simulink model "Tischpendel"  (R2014a)
settings: Solver=ode45  StartTime=0.0  StopTime=1000  RelTol=1e-3
libraries: simulink x1
settings Model: Creator=Anton  LastModifiedBy=hollowman
settings DebuggingCC: UnderspecifiedInitializationDetection=Classic

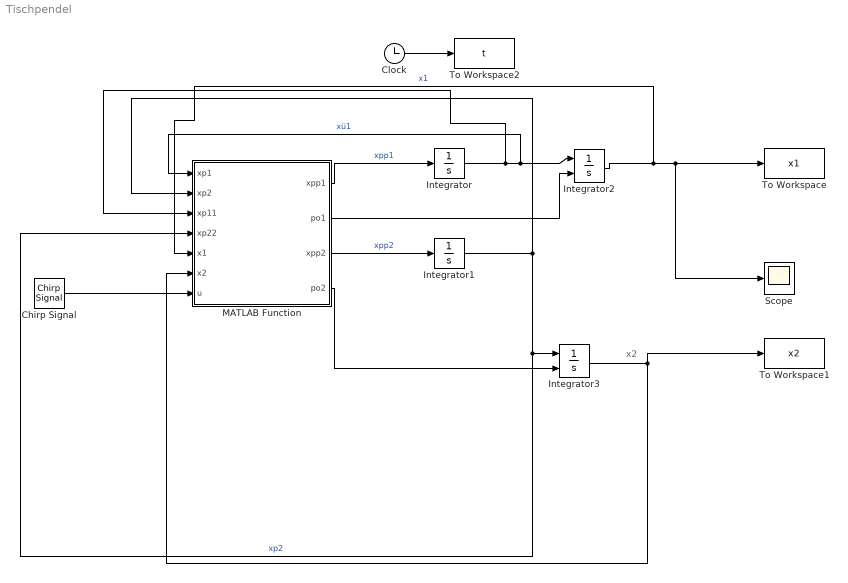
== system Tischpendel ==
  note: x2
  Chirp Signal : simulink/Sources/Chirp Signal  f1=0.5  T=100  f2=100
  Clock : Clock
  Integrator : Integrator
  Integrator1 : Integrator
  Integrator2 : Integrator  InitialConditionSource=external
  Integrator3 : Integrator  InitialConditionSource=external
  MATLAB Function : MATLAB Function  TreatAsAtomicUnit=on
  Scope : Scope
      settings: TimeRange=5  YMin=-2e+195  YMax=1e+195
  To Workspace : ToWorkspace  VariableName=x1  SampleTime=-1
  To Workspace1 : ToWorkspace  VariableName=x2  SampleTime=-1
  To Workspace2 : ToWorkspace  VariableName=t  SampleTime=-1
  wires:
  Integrator3/1 -> To Workspace1/1, MATLAB Function/6(x2)
  Integrator2/1 -> MATLAB Function/5(x1), Scope/1, To Workspace/1  "x1"
  Clock/1 -> To Workspace2/1
  Integrator/1 -> MATLAB Function/3(xp11), MATLAB Function/1(xp1), Integrator2/1  "xü1"
  MATLAB Function/1(xpp1) -> Integrator/1  "xpp1"
  Chirp Signal/1 -> MATLAB Function/7(u)
  MATLAB Function/3(xpp2) -> Integrator1/1  "xpp2"
  Integrator1/1 -> MATLAB Function/4(xp22), Integrator3/1, MATLAB Function/2(xp2)  "xp2"
  MATLAB Function/2(po1) -> Integrator2/2
  MATLAB Function/4(po2) -> Integrator3/2

== matlab function Tischpendel/MATLAB Function ==
  data: xp1 input; xp2 input; xp11 input; xp22 input; x1 input; x2 input; u input; xpp1 output; po1 output; xpp2 output; po2 output
function [xpp1, po1, xpp2, po2] = fcn(xp1,xp2,xp11,xp22,x1,x2,u)
c1 = 15000;    %[N/m]
c2 = 10000;     %[N/m]
m1 = 60;        %kg
m2 = 450;       %kg
d = 600;        %Ns/m
g = 9.81;       %m/s^2

Fc = (u-x1)*c1;       %Federkraft
Fd =  d * (xp2-xp1);  %Wiederstandskraft

xpp1 = (2 *(Fc + Fd)-(m1 * g))/m1;

Fc2 = (u-x2)*c2;
Fd2 = d * (xp22-xp11);

xpp2 = (2*(Fc2 - Fd2)-(m2 * g))/m2;

po1 = 2 *(Fc) - (m1  * g);
po2 = 2 *(Fc2) - (m2  * g);
